simulink model "SimulinkR"  (R2022b)
settings: Solver=VariableStepAuto  StartTime=0.0  StopTime=30.0  RelTol=1e-3
values from neighbouring files (symbols this model uses):
  A = [0 1 0 0 0 0; A1 0 0 0 A2 0; 0 0 0 1 0 0; A3 0 0 0 A4 0; 0 0 0 0 0 1; A5 0 0 0 A6 0]    [LQRFun.m]    (also in jisuan.m = [2 1;-4 2])
  B = [0 0; B1 B2; 0 0; B3 B4; 0 0; B5 B6]    [LQRFun.m]
  C = eye(6,6)    [LQRFun.m]
  D = eye(6,2)    [LQRFun.m]
  K = lqr(A,B,MatQ,MatR)    [LQRFun.m]    (also in WBliteLQR.m = LQRFun(BasicData,ValData,Q,R); WBliteLQR2.m = LQRFun(BasicData,ValData,Q,R); WBliteLQR3.m = LQRFun(BasicData,ValData,Q,R); WBliteLQR4.m = LQRFun(BasicData,ValData,Q_leg,R_leg))
undefined symbols (not defined in the file or in its folder): ConstA, Continuous, Time, X0
libraries: ctrlSharedLib x1
settings Model: Creator=qianw  LastModifiedBy=qianw
settings OptimizationCC: DefaultParameterBehavior=Inlined  UseDivisionForNetSlopeComputation=on  GainParamInheritBuiltInType=on  UseFloatMulNetSlope=on  InlineInvariantSignals=on  EfficientFloat2IntCast=on  LifeSpan=1
settings HardwareCC: ProdLongLongMode=on  ProdHWDeviceType=AMD->x86-64 (Windows64)
settings SFSimCC: MATLABDynamicMemAlloc=off
settings RTWCC: GenerateReport=on  LaunchReport=on
settings CodeAppCC: ForceParamTrailComments=on
settings GRTTargetCC: CombineSignalStateStructs=on  MatFileLogging=off  SupportVariableSizeSignals=on

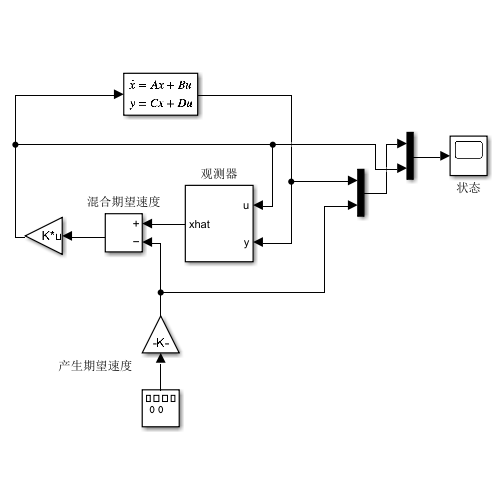
[thumbnail: Simulink's stored preview of the top-level diagram]
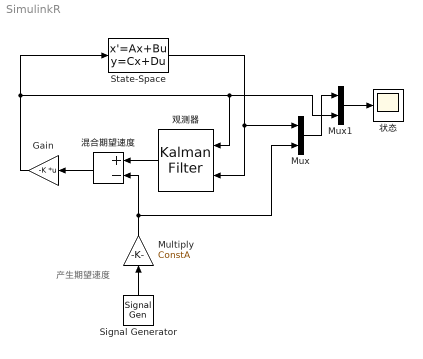
== system SimulinkR ==
  note: 产生期望速度
  Gain : Gain  Gain=-K  Multiplication=Matrix(K*u)
  Multiply : Gain  Gain=ConstA
  Mux : Mux  Inputs=2
  Mux1 : Mux  Inputs=2
  Signal Generator : SignalGenerator  Units=rad/sec
  State-Space : StateSpace  A=A  B=B  C=C  D=D  InitialCondition=X0
  混合期望速度 : Sum  Inputs=+-
  状态 : Scope
  观测器 : ctrlSharedLib/Kalman Filter  TimeDomain=Continuous-Time  UseCurrentEstimator=on  ModelSource=Individual A, B, C, D matrices  ModelSourceVariable=ss(0.95,1,1,0,1)  A=A  B=B  C=C  D=D  NumberOfStates=1  NumberOfInputs=1  NumberOfOutputs=1  InitialEstimateSource=Dialog  X0=0  P0=10  UseK=off  UseGH=off  NumberOfProcessNoiseInputs=1  G=1  TimeInvariantG=on  H=0  TimeInvariantH=on  Q=0.05  TimeInvariantQ=on  R=1  TimeInvariantR=on  N=0  TimeInvariantN=on  AddInputPort=on  AddEnablePort=off  OutputEstimatedY=off  OutputP=off  Ts=-1
  wires:
  State-Space/1 -> Mux/1, 观测器/2
  Gain/1 -> State-Space/1, Mux1/2, 观测器/1
  混合期望速度/1 -> Gain/1
  观测器/1 -> 混合期望速度/1
  Signal Generator/1 -> Multiply/1
  Multiply/1 -> 混合期望速度/2, Mux/2
  Mux1/1 -> 状态/1
  Mux/1 -> Mux1/1
